simulink model "gm_PN_generatorV2_interface_tx"  (R2020a)
settings: Solver=FixedStepDiscrete  StartTime=0.0  StopTime=20  RelTol=1e-3  EnableMultiTasking=on
undefined symbols (not defined in the file): AXI4, Lite
libraries: axiinterfacelib x3, commfilt2 x2, commchan3 x1, commdigbbndpm3 x1
settings Model: Creator=juanj  LastModifiedBy=juanj
settings SolverCC: PositivePriorityOrder=on
settings OptimizationCC: BlockReduction=off  ConditionallyExecuteInputs=off  EnhancedBackFolding=on  PassReuseOutputArgsAs=Individual arguments  ZeroExternalMemoryAtStartup=off  ZeroInternalMemoryAtStartup=off  MaxStackSize=64  OptimizeBlockOrder=speed  DifferentSizesBufferReuse=on  OptimizationCustomize=off  EfficientTunableParamExpr=on
settings DebuggingCC: AlgebraicLoopMsg=error  SingleTaskRateTransMsg=error  ParameterTunabilityLossMsg=error
settings HardwareCC: ProdBitPerPointer=32  ProdBitPerSizeT=32  ProdBitPerPtrDiffT=32  ProdLargestAtomicInteger=Long  ProdLargestAtomicFloat=Double  ProdWordSize=32  ProdLongLongMode=on  ProdHWDeviceType=ARM Compatible->ARM Cortex  TargetBitPerPointer=64  TargetBitPerSizeT=64  TargetBitPerPtrDiffT=64  TargetLongLongMode=on  TargetIntDivRoundTo=Zero  TargetEndianess=LittleEndian  TargetWordSize=64  TargetHWDeviceType=Custom Processor->MATLAB Host Computer
settings SFSimCC: MATLABDynamicMemAlloc=off
settings RTWCC: SystemTargetFile=ert.tlc  HardwareBoard=ZedBoard  TemplateMakefile=ert_default_tmf  Toolchain=Linaro AArch32 Linux v6.3.1
settings CodeAppCC: ForceParamTrailComments=on  IgnoreCustomStorageClasses=off  OperatorAnnotations=on  SimulinkDataObjDesc=on  SFDataObjDesc=on  InsertBlockDesc=on

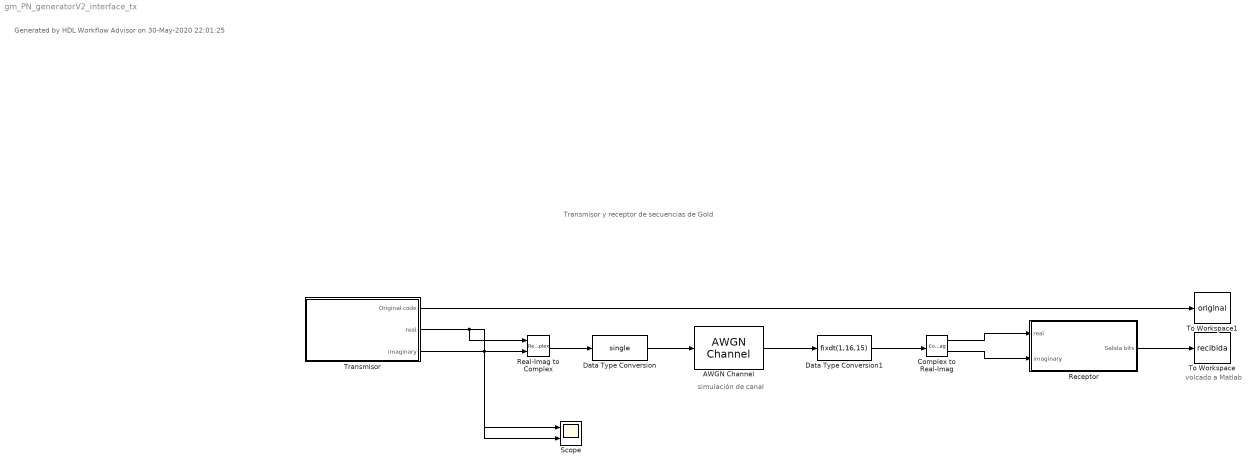
== system gm_PN_generatorV2_interface_tx ==
  note: Transmisor y receptor de secuencias de Gold
  note: simulación de canal
  note: volcado a Matlab
  note: Generated by HDL Workflow Advisor on 30-May-2020 22:01:25
  AWGN Channel : commchan3/AWGN Channel  InputProcessing=Columns as channels (frame based)  seed=67  noiseMode="Signal to noise ratio  (Es/No)"  EbNodB=10  EsNodB=10  SNRdB=10  bitsPerSym=1  Ps=1  Tsym=0.1  variance=1
  Complex to Real-Imag : ComplexToRealImag
  Data Type Conversion : DataTypeConversion  OutDataTypeStr=single
  Data Type Conversion1 : DataTypeConversion  OutDataTypeStr=fixdt(1,16,15)
  Real-Imag to Complex : RealImagToComplex
  Receptor : Subsystem  TreatAsAtomicUnit=on
  Scope : Scope  NumInputPorts=2
  To Workspace : ToWorkspace  VariableName=recibida  SampleTime=-1
      settings: Save2DSignal=2-D array (concatenate along first dimension)
  To Workspace1 : ToWorkspace  VariableName=original  SampleTime=-1
      settings: Save2DSignal=2-D array (concatenate along first dimension)
  Transmisor : Subsystem  TreatAsAtomicUnit=on  mask(AXI4-Lite/AXI4 Interface){}
      mask help:
      | This is an automatically generated subsystem block.
      | This contains the AXI interface blocks that communicate with the PN_genera_ip_tx IPCore generated from PN_generatorV2/Transmisor subsystem.
      mask Display: disp(sprintf('Xilinx Zynq \nAXI Interface'));
  wires:
  Transmisor/1(Original code) -> To Workspace1/1
  Data Type Conversion/1 -> AWGN Channel/1
  Data Type Conversion1/1 -> Complex to Real-Imag/1
  AWGN Channel/1 -> Data Type Conversion1/1
  Complex to Real-Imag/2 -> Receptor/2(imaginary)
  Complex to Real-Imag/1 -> Receptor/1(real)
  Transmisor/2(real) -> Real-Imag to Complex/1, Scope/1
  Transmisor/3(imaginary) -> Real-Imag to Complex/2, Scope/2
  Real-Imag to Complex/1 -> Data Type Conversion/1
  Receptor/1(Salida bits) -> To Workspace/1

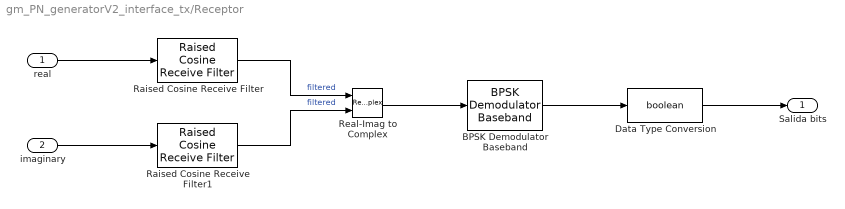
== system gm_PN_generatorV2_interface_tx/Receptor ==
  real : Inport
  imaginary : Inport  Port=2
  BPSK Demodulator Baseband : commdigbbndpm3/BPSK Demodulator Baseband  DecType=Hard decision  VarSource=Dialog  Variance=1  Ph=0  outDtype=Inherit via internal rule  derotateFactorWordLen=16  derotateFactorDataTypeStr=Inherit: Same word length as input  derotateFactorLastDataTypeStr=Inherit: Same word length as input
  Data Type Conversion : DataTypeConversion  OutDataTypeStr=boolean
  Raised Cosine Receive Filter : commfilt2/Raised Cosine Receive Filter  filtType=Square root  R=0.5  filtSpan=16  N=16  downFactor=16  downOffset=0  filterGain=2  RateOptions=Allow multirate processing  framing=Mute  checkCoeff=off  variableName=rcRxFilt  currentFiltSpan=16  D=(16)/2  inputOffset=0  sampMode=Mute  saveAsFlag=0  rateMode=Downsampling  checkGain=Normalized  launchFVT=on  roundingMode=Floor  overflowMode=off  coeffDataTypeStr=Inherit: Same word length as input  coeffMin=[]  coeffMax=[]  coeffLastDataTypeStr=Inherit: Same word length as input  accumDataTypeStr=Inherit: Same as product output  accumLastDataTypeStr=Inherit: Same as product output  outputDataTypeStr=Inherit: Same as accumulator  outputMin=[]  outputMax=[]  outputLastDataTypeStr=Inherit: Same as accumulator
  Raised Cosine Receive Filter1 : commfilt2/Raised Cosine Receive Filter  filtType=Square root  R=0.5  filtSpan=16  N=16  downFactor=16  downOffset=0  filterGain=2  RateOptions=Allow multirate processing  framing=Mute  checkCoeff=off  variableName=rcRxFilt1  currentFiltSpan=16  D=(16)/2  inputOffset=0  sampMode=Mute  saveAsFlag=0  rateMode=Downsampling  checkGain=Normalized  launchFVT=on  roundingMode=Floor  overflowMode=off  coeffDataTypeStr=Inherit: Same word length as input  coeffMin=[]  coeffMax=[]  coeffLastDataTypeStr=Inherit: Same word length as input  accumDataTypeStr=Inherit: Same as product output  accumLastDataTypeStr=Inherit: Same as product output  outputDataTypeStr=Inherit: Same as accumulator  outputMin=[]  outputMax=[]  outputLastDataTypeStr=Inherit: Same as accumulator
  Real-Imag to Complex : RealImagToComplex
  Salida bits : Outport
  wires:
  Data Type Conversion/1 -> Salida bits/1
  real/1 -> Raised Cosine Receive Filter/1
  Real-Imag to Complex/1 -> BPSK Demodulator Baseband/1
  Raised Cosine Receive Filter1/1 -> Real-Imag to Complex/2  "filtered"
  imaginary/1 -> Raised Cosine Receive Filter1/1
  BPSK Demodulator Baseband/1 -> Data Type Conversion/1
  Raised Cosine Receive Filter/1 -> Real-Imag to Complex/1  "filtered"

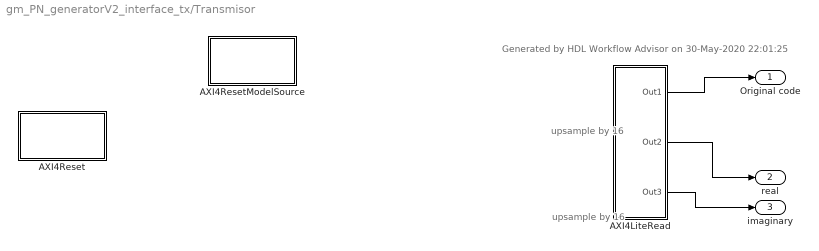
== system gm_PN_generatorV2_interface_tx/Transmisor ==
  note: upsample by 16
  note: upsample by 16
  note: Generated by HDL Workflow Advisor on 30-May-2020 22:01:25
  AXI4LiteRead : Subsystem  Priority=10
  AXI4Reset : Subsystem  mask(System Start){ShowInLibBrowser=0}
      mask prompts: ShowInLibBrowser "Simulink:masks:CustCodeMaskParam1_MP"
      settings: CopyFcn=cccopyfcn(gcb)  OpenFcn=ccopenfcn('System Start Function')
      mask Help: eval('feval(''rtwprivate'',''rtwhelpview'',''rtw_sys_start_block'')');
      mask Display: disp('System\nStart');
  AXI4ResetModelSource : Subsystem  mask(Model Source){ShowInLibBrowser=0}
      mask prompts: ShowInLibBrowser "Simulink:masks:CustCodeMaskParam1_MP"
      settings: CopyFcn=cccopyfcn(gcb)  OpenFcn=ccopenfcn('Model Source')
      mask Help: eval('feval(''rtwprivate'',''rtwhelpview'',''rtw_model_source_block'')');
      mask Display: disp('Model\nSource');
  Original code : Outport
  real : Outport  Port=2
  imaginary : Outport  Port=3
  wires:
  AXI4LiteRead/1(Out1) -> Original code/1
  AXI4LiteRead/2(Out2) -> real/1
  AXI4LiteRead/3(Out3) -> imaginary/1

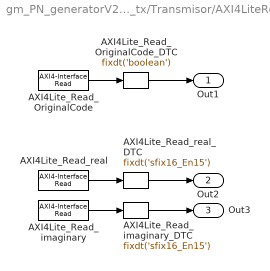
== system gm_PN_generatorV2_interface_tx/Transmisor/AXI4LiteRead ==
  AXI4Lite_Read_OriginalCode : axiinterfacelib/AXI4-Interface Read  Priority=2  AXIInterfaceType=AXI4-Lite  DeviceName=/dev/mwipcore  RegisterOffset=hex2dec('100')  DataLength=1  DataType=uint32  SampleTime=-1  blockPlatform=ZYNQ  SimulateUsing=Interpreted Execution
      settings: SourceProductBaseCode=ECZYNQ7000
  AXI4Lite_Read_OriginalCode_DTC : DataTypeConversion  OutDataTypeStr=fixdt('boolean')  ConvertRealWorld=Stored Integer (SI)
  AXI4Lite_Read_imaginary : axiinterfacelib/AXI4-Interface Read  Priority=4  AXIInterfaceType=AXI4-Lite  DeviceName=/dev/mwipcore  RegisterOffset=hex2dec('108')  DataLength=1  DataType=uint32  SampleTime=-1  blockPlatform=ZYNQ  SimulateUsing=Interpreted Execution
      settings: SourceProductBaseCode=ECZYNQ7000
  AXI4Lite_Read_imaginary_DTC : DataTypeConversion  OutDataTypeStr=fixdt('sfix16_En15')  ConvertRealWorld=Stored Integer (SI)
  AXI4Lite_Read_real : axiinterfacelib/AXI4-Interface Read  Priority=3  AXIInterfaceType=AXI4-Lite  DeviceName=/dev/mwipcore  RegisterOffset=hex2dec('104')  DataLength=1  DataType=uint32  SampleTime=-1  blockPlatform=ZYNQ  SimulateUsing=Interpreted Execution
      settings: SourceProductBaseCode=ECZYNQ7000
  AXI4Lite_Read_real_DTC : DataTypeConversion  OutDataTypeStr=fixdt('sfix16_En15')  ConvertRealWorld=Stored Integer (SI)
  Out1 : Outport
  Out2 : Outport  Port=2
  Out3 : Outport  Port=3
  wires:
  AXI4Lite_Read_real/1 -> AXI4Lite_Read_real_DTC/1
  AXI4Lite_Read_imaginary_DTC/1 -> Out3/1
  AXI4Lite_Read_imaginary/1 -> AXI4Lite_Read_imaginary_DTC/1
  AXI4Lite_Read_OriginalCode/1 -> AXI4Lite_Read_OriginalCode_DTC/1
  AXI4Lite_Read_real_DTC/1 -> Out2/1
  AXI4Lite_Read_OriginalCode_DTC/1 -> Out1/1

== system gm_PN_generatorV2_interface_tx/Transmisor/AXI4Reset ==

== system gm_PN_generatorV2_interface_tx/Transmisor/AXI4ResetModelSource ==
